simulink model "example_CollectorEN12975"  (R2013b)
settings: Solver=ode45  StartTime=0.0  StopTime=24*3600  MaxStep=1800  RelTol=1e-3
libraries: carnot x6
settings Model: Creator=drhf  LastModifiedBy=drhf
settings OptimizationCC: ExpressionDepthLimit=2147483647
settings DebuggingCC: StateNameClashWarn=warning
settings GRTTargetCC: CombineOutputUpdateFcns=off  GRTInterface=on

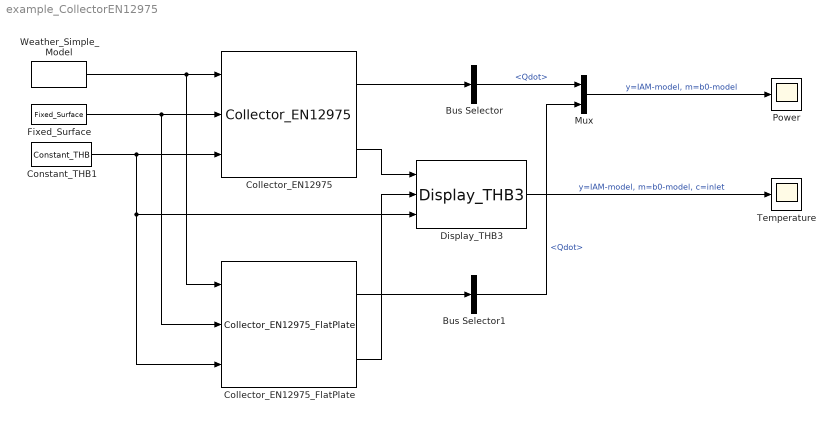
== system example_CollectorEN12975 ==
  Bus Selector : BusSelector  OutputSignals=Qdot
  Bus Selector1 : BusSelector  OutputSignals=Qdot
  Collector_EN12975 : carnot/Source/Solar_Thermal/Collector_EN12975  acol=2.5  len=2.3  fta=0.8103  c1=3.757  c2=0.0147  c3=0  c4=0  c5=7062  c6=0  kblangle=[0:5:90]  KbL="[1.0000    1.0000    0.9999    0.9996    0.9991    0.9982    0.9965  0.9935    0.9886    0.9807    0.9678    0.9473    0.9148    0.8638   0.7846    0.6644    0.4907    0.2599    0.0000]"  kbtangle=[0:5:90]  KbT=[1.00000 1.00000 1.00000 1.00000 1.00000 1.00000 1.00000 1.00000 1.00000 1.00000 1.00000 0.87500 0.75000 0.62500 0.50000 0.37500 0.25000 0.12500 0]  Kd=0.92  lin=0  qua=0  tini=20
  Collector_EN12975_FlatPlate : carnot/Source/Solar_Thermal/Collector_EN12975_FlatPlate  acol=2.5  len=2.3  fta=0.8103  c1=3.757  c2=0.0147  c3=0  c4=0  c5=7062  c6=0  b0=0.12  Kd=0.92  lin=0  qua=0  tini=20
  Constant_THB1 : carnot/Source/Simple/Constant_THB  t=40  mdot=100/3600  p=1e5  mID=No Pressure Drop  fluid=Water  mix=0  dia=0.02  hgt=0
  Display_THB3 : carnot/Outputs/Display_THB3  t=on  m=off  p=off  id=off  mix=off  d=off
  Fixed_Surface : carnot/Weather/Fixed_Surface  colangle=30  colazi=0  colrot=0
  Mux : Mux  Inputs=2
  Power : Scope
  Temperature : Scope
  Weather_Simple_Model : carnot/Weather/Weather_Simple_Model  lat=60  Ibn=900  Idg=100  tamb=5  deltaTsky=-6  rh=50  precip="10e-3/24/3600           % 10 mm in 24 h"  cloud=0.125  p=1013e2  vw=1  wdir=270
  wires:
  Weather_Simple_Model/1 -> Collector_EN12975/1, Collector_EN12975_FlatPlate/1
  Fixed_Surface/1 -> Collector_EN12975/2, Collector_EN12975_FlatPlate/2
  Constant_THB1/1 -> Collector_EN12975/3, Collector_EN12975_FlatPlate/3, Display_THB3/3
  Collector_EN12975/2 -> Display_THB3/1
  Display_THB3/1 -> Temperature/1  "y=IAM-model, m=b0-model, c=inlet"
  Collector_EN12975_FlatPlate/2 -> Display_THB3/2
  Collector_EN12975/1 -> Bus Selector/1
  Collector_EN12975_FlatPlate/1 -> Bus Selector1/1
  Bus Selector/1 -> Mux/1  "<Qdot>"
  Bus Selector1/1 -> Mux/2  "<Qdot>"
  Mux/1 -> Power/1  "y=IAM-model, m=b0-model"
